simulink model "tmpmatching"  (Simulink 7.5)
settings: Solver=VariableStepDiscrete  StartTime=0.0  StopTime=570  RelTol=1e-3
undefined symbols (not defined in the file or in its folder): gray, Rec, SDTV
libraries: vipconversions x1, viptextngfix x1, dspsrcs4 x1, vipsrcs x1, vipanalysis x1, dspsnks4 x1, vipsnks x1
settings Model: Creator=lengoanhcat  LastModifiedBy=lengoanhcat

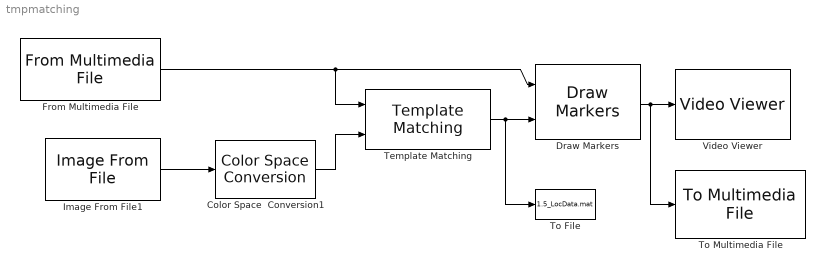
== system tmpmatching ==
  Color Space  Conversion1 : vipconversions/Color Space  Conversion  conversion=Obsolete  conversionActive=R'G'B' to intensity  wp_str=D65  rec=Rec. 601 (SDTV)  sys=1125/60/2:1  imagePorts=One multidimensional signal
  Draw Markers : viptextngfix/Draw Markers  DialogController=vipDDGCreate  DialogControllerArgs=DataTag0  shape=X-mark  size=10  fill=off  fillClrSource=Specify via dialog  display=Black  intensity=200  color=[200 255 100]  opacity=0.6  viewport=Entire image  antialiasing=off  inType=Obsolete  imagePorts=One multidimensional signal  prodOutputMode=Binary point scaling  prodOutputWordLength=32  prodOutputFracLength=14  memoryMode=Specify word length  memoryWordLength=16  memoryFracLength=15  roundingMode=Floor  overflowMode=off
  From Multimedia File : dspsrcs4/From Multimedia File  DialogController=dspDDGCreate  DialogControllerArgs=DataTag1  inputFilename=C:\Users\lengoanhcat\Documents\MATLAB\Experiment_8\template_matching\1.5.mp4  loop=on  numPlays=1  outputStreams=Video only  videoDataType=single  audioDataType=int16  inheritSampleTime=on  userDefinedSampleTime=1/30  noAudioOutput=off  isIntensityVideo=off  fourcc=Intensity  colorVideoFormat=One multidimensional signal  outputEOF=off  dataOrg=Column-major  audioFrameSize=1024  computeAudioFrameSize=off
  Image From File1 : vipsrcs/Image From File  Tag=vipblks_nd  DialogController=vipDDGCreate  DialogControllerArgs=DataTag2  SystemSampleTime=-1  FileName=C:\Users\lengoanhcat\Documents\MATLAB\Experiment_8\template_matching\template.jpg  imagePorts=One multidimensional signal  Ts=inf  ImageDataType=single  Signed=on  WordLength=16  sdImageDataType=uint(8)  FractionLengthMode=User-defined  FractionLength=15  OutPortLabels=R|G|B
  Template Matching : vipanalysis/Template Matching  DialogController=vipDDGCreate  DialogControllerArgs=DataTag3  metric=Maximum absolute difference  output=Best match location  method=Exhaustive  nMetric=off  nSize=3  roi=off  roiValid=off  accumMode=Binary point scaling  accumWordLength=32  accumFracLength=0  prodOutputMode=Binary point scaling  prodOutputWordLength=32  prodOutputFracLength=0  roundingMode=Floor  overflowMode=off
  To File : ToFile  Filename=1.5_LocData.mat  MatrixName=Loc  SaveFormat=Timeseries
  To Multimedia File : dspsnks4/To Multimedia File  DialogController=dspDDGCreate  DialogControllerArgs=DataTag4  outputFilename=C:\Users\lengoanhcat\Documents\MATLAB\Experiment_8\template_matching\video_tracked.avi  streamSelection=Video only  videoCompressor=None (uncompressed)  audioCompressor=None (uncompressed)  imagePorts=One multidimensional signal  fileType=AVI  audioDatatype=Determine from input data type  fourcc=RGB
  Video Viewer : vipsnks/Video Viewer  DialogControllerArgs=DataTag6  inputType=Obsolete7b  imagePorts=One multidimensional signal  useColorMap=off  colormapValue=gray(256)  specRange=off  minInputVal=0  maxInputVal=255  FigPos=[184 881 899 693]  AxisZoom=on  trueSizedOnce=off  OpenAtMdlStart=on
  wires:
  Template Matching/1 -> Draw Markers/2, To File/1
  Draw Markers/1 -> Video Viewer/1, To Multimedia File/1
  Color Space  Conversion1/1 -> Template Matching/2
  Image From File1/1 -> Color Space  Conversion1/1
  From Multimedia File/1 -> Template Matching/1, Draw Markers/1
